simulink model "PosControl_Sim"  (R2016b)
settings: Solver=ode4  StartTime=0.0  StopTime=20  FixedStep=0.001  RelTol=1e-3
InitFcn:
  | Init_control;
values from neighbouring files (symbols this model uses):
  DEG2RAD = 0.0174533    [Init_control.m]
  Kd_PITCH_AgngleRate = 0.001    [Init_control.m]
  Kd_ROLL_AgngleRate = 0.001    [Init_control.m]
  Kd_YAW_AngleRate = 0.00    (= 0)    [Init_control.m]
  Ki_PITCH_AgngleRate = 0.02    [Init_control.m]
  Ki_ROLL_AgngleRate = 0.02    [Init_control.m]
  Ki_YAW_AngleRate = 0.01    [Init_control.m]
  Kp_PITCH_AgngleRate = 0.1    [Init_control.m]
  Kp_PITCH_ANGLE = 6.5    [Init_control.m]
  Kp_ROLL_AgngleRate = 0.1    [Init_control.m]
  Kp_ROLL_ANGLE = 6.5    [Init_control.m]
  Kp_YAW_AngleRate = 0.3    [Init_control.m]
  Kpxp = 1.2    [Init_control.m]
  Kpyp = 1.2    [Init_control.m]
  Kpzp = 4.0    (= 4)    [Init_control.m]
  Kvxd = 0.01    [Init_control.m]
  Kvxi = 0.4    [Init_control.m]
  Kvxp = 1.5    [Init_control.m]
  Kvyd = 0.01    [Init_control.m]
  Kvyi = 0.4    [Init_control.m]
  Kvyp = 1.5    [Init_control.m]
  Kvzd = 0.005    [Init_control.m]
  Kvzi = 0.01    [Init_control.m]
  Kvzp = 0.45    [Init_control.m]
  MAX_CONTROL_ANGLE_PITCH = 35    [Init_control.m]
  MAX_CONTROL_ANGLE_RATE_PITCH = 220    [Init_control.m]
  MAX_CONTROL_ANGLE_RATE_ROLL = 220    [Init_control.m]
  MAX_CONTROL_ANGLE_RATE_Y = 200    [Init_control.m]
  MAX_CONTROL_ANGLE_ROLL = 35    [Init_control.m]
  MAX_CONTROL_VELOCITY_XY = 5    [Init_control.m]
  MAX_CONTROL_VELOCITY_Z = 3    [Init_control.m]
  MAX_MAN_THR = 0.9    [Init_control.m]
  Saturation_I_ah = 3.43    [Init_control.m]
  Saturation_I_az = 5    [Init_control.m]
  Saturation_I_RP_Max = 0.3    [Init_control.m]
  Saturation_I_RP_Min = -0.3    [Init_control.m]
  Saturation_I_Y_Max = 0.2    [Init_control.m]
  Saturation_I_Y_Min = -0.2    [Init_control.m]
  THR_HOVER = 0.6085    [Init_control.m]
undefined symbols (not defined in the file or in its folder): DiscIntNeverNeededParam, earthRadius, ModelInit_RPM, ModelParam_envGravityAcc, ModelParam_motorCr, ModelParam_motorJm, ModelParam_motorT, ModelParam_motorWb, ModelParam_rotorCm, ModelParam_rotorCt, ModelParam_uavCd, ModelParam_uavJ, ModelParam_uavMass, ModelParam_uavR
libraries: simulink x7, aerolibutil x2, aerolibfltsims x2, aerolibtransform2 x1, aerolibanimutils x1
settings Model: Creator=dream  LastModifiedBy=Mr Wang
settings DebuggingCC: BusObjectLabelMismatch=error

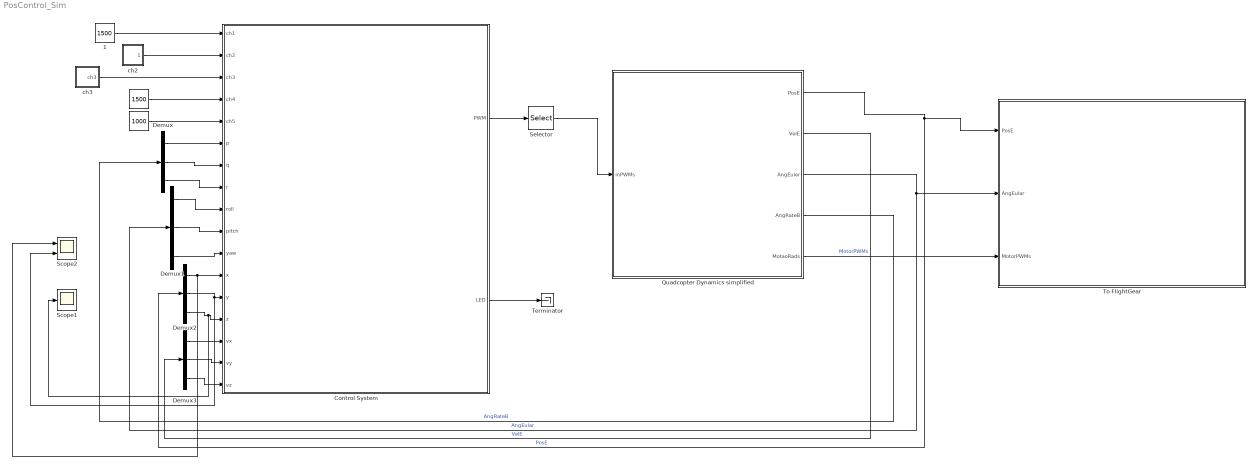
== system PosControl_Sim ==
  " " : Constant  Value=1000  OutDataTypeStr=uint16
  "          " : Constant  Value=1500  OutDataTypeStr=uint16
  "   1" : Constant  Value=1500  OutDataTypeStr=uint16
  Control System : Subsystem
      mask Display: image('icon\pixhawk.png');
  Demux{,1..3} (4 alike) : Demux  Outputs=3
  "Quadcopter Dynamics simplified " : Subsystem
      mask Display: image('./icon/F450.png');
  Scope1 : Scope
  Scope2 : Scope  NumInputPorts=2
  Selector : Selector  InputPortWidth=8  IndexOptions=Index vector (dialog)  Indices=[1:4]  OutputSizes=1
  Terminator : Terminator
  To FlightGear : Subsystem
      mask Display: image('./icon/FlightGear.png');
  ch2 : Subsystem
  ch3 : Subsystem
  wires:
  "Quadcopter Dynamics simplified "/1(PosE) -> To FlightGear/1(PosE), Demux2/1  "PosE"
  "Quadcopter Dynamics simplified "/5(MotaoRads) -> To FlightGear/3(MotorPWMs)  "MotorPWMs"
  Control System/2(LED) -> Terminator/1
  "Quadcopter Dynamics simplified "/3(AngEuler) -> To FlightGear/2(AngEular), Demux1/1  "AngEular"
  "          "/1 -> Control System/4(ch4)
  "Quadcopter Dynamics simplified "/4(AngRateB) -> Demux/1  "AngRateB"
  " "/1 -> Control System/5(ch5)
  Demux/1 -> Control System/6(p)
  Demux/2 -> Control System/7(q)
  Demux/3 -> Control System/8(r)
  Demux1/1 -> Control System/9(roll)
  Demux1/2 -> Control System/10(pitch)
  Demux1/3 -> Control System/11(yaw)
  Control System/1(PWM) -> Selector/1
  Demux2/1 -> Control System/12(x), Scope2/1
  Demux2/2 -> Scope2/2, Control System/13(y)
  Demux2/3 -> Scope1/1, Control System/14(z)
  Demux3/1 -> Control System/15(vx)
  Demux3/2 -> Control System/16(vy)
  Demux3/3 -> Control System/17(vz)
  "Quadcopter Dynamics simplified "/2(VelE) -> Demux3/1  "VelE"
  "   1"/1 -> Control System/1(ch1)
  ch2/1(ch2) -> Control System/2(ch2)
  ch3/1(ch3) -> Control System/3(ch3)
  Selector/1 -> "Quadcopter Dynamics simplified "/1(inPWMs)

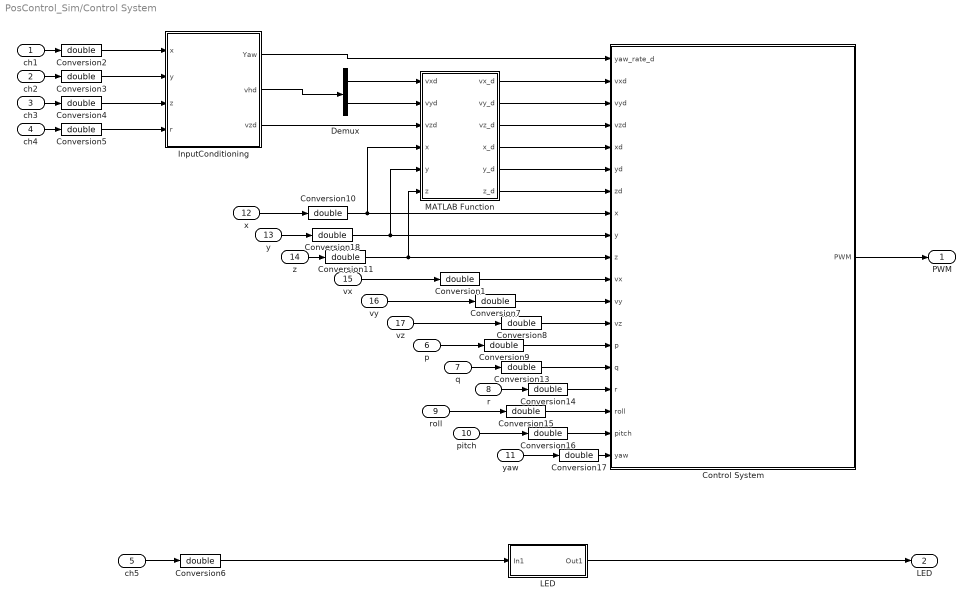
== system PosControl_Sim/Control System ==
  ch1 : Inport  OutDataTypeStr=uint16  PortDimensions=1
  ch2 : Inport  Port=2  OutDataTypeStr=uint16  PortDimensions=1
  ch3 : Inport  Port=3  OutDataTypeStr=uint16  PortDimensions=1
  ch4 : Inport  Port=4  OutDataTypeStr=uint16  PortDimensions=1
  ch5 : Inport  Port=5  OutDataTypeStr=uint16  PortDimensions=1  Interpolate=off
  p : Inport  Port=6  PortDimensions=1
  q : Inport  Port=7  PortDimensions=1
  r : Inport  Port=8  PortDimensions=1
  roll : Inport  Port=9  PortDimensions=1
  pitch : Inport  Port=10  PortDimensions=1
  yaw : Inport  Port=11  PortDimensions=1
  x : Inport  Port=12
  y : Inport  Port=13
  z : Inport  Port=14
  vx : Inport  Port=15
  vy : Inport  Port=16
  vz : Inport  Port=17
  Control System : Subsystem
  Conversion{1..11,13..18} (17 alike) : DataTypeConversion  OutDataTypeStr=double
  Demux : Demux  Outputs=2
  InputConditioning : Subsystem
  "LED " : Subsystem
  MATLAB Function : MATLAB Function  TreatAsAtomicUnit=on
  PWM : Outport  PortDimensions=8
  LED : Outport  Port=2  PortDimensions=1
  wires:
  ch3/1 -> Conversion4/1
  ch5/1 -> Conversion6/1
  InputConditioning/1(Yaw) -> Control System/1(yaw_rate_d)
  ch4/1 -> Conversion5/1
  "LED "/1(Out1) -> LED/1
  Conversion6/1 -> "LED "/1(In1)
  Conversion5/1 -> InputConditioning/4(r)
  Control System/1(PWM) -> PWM/1
  ch1/1 -> Conversion2/1
  ch2/1 -> Conversion3/1
  InputConditioning/2(vhd) -> Demux/1
  Demux/1 -> MATLAB Function/1(vxd)
  Demux/2 -> MATLAB Function/2(vyd)
  InputConditioning/3(vzd) -> MATLAB Function/3(vzd)
  y/1 -> Conversion18/1
  z/1 -> Conversion11/1
  vy/1 -> Conversion7/1
  MATLAB Function/4(x_d) -> Control System/5(xd)
  MATLAB Function/5(y_d) -> Control System/6(yd)
  MATLAB Function/6(z_d) -> Control System/7(zd)
  Conversion2/1 -> InputConditioning/1(x)
  Conversion3/1 -> InputConditioning/2(y)
  vx/1 -> Conversion1/1
  Conversion1/1 -> Control System/11(vx)
  Conversion7/1 -> Control System/12(vy)
  vz/1 -> Conversion8/1
  Conversion8/1 -> Control System/13(vz)
  Conversion18/1 -> MATLAB Function/5(y), Control System/9(y)
  Conversion11/1 -> MATLAB Function/6(z), Control System/10(z)
  MATLAB Function/1(vx_d) -> Control System/2(vxd)
  MATLAB Function/2(vy_d) -> Control System/3(vyd)
  MATLAB Function/3(vz_d) -> Control System/4(vzd)
  roll/1 -> Conversion15/1
  pitch/1 -> Conversion16/1
  p/1 -> Conversion9/1
  q/1 -> Conversion13/1
  r/1 -> Conversion14/1
  Conversion9/1 -> Control System/14(p)
  Conversion13/1 -> Control System/15(q)
  Conversion14/1 -> Control System/16(r)
  Conversion15/1 -> Control System/17(roll)
  Conversion16/1 -> Control System/18(pitch)
  yaw/1 -> Conversion17/1
  Conversion17/1 -> Control System/19(yaw)
  Conversion4/1 -> InputConditioning/3(z)
  x/1 -> Conversion10/1
  Conversion10/1 -> MATLAB Function/4(x), Control System/8(x)

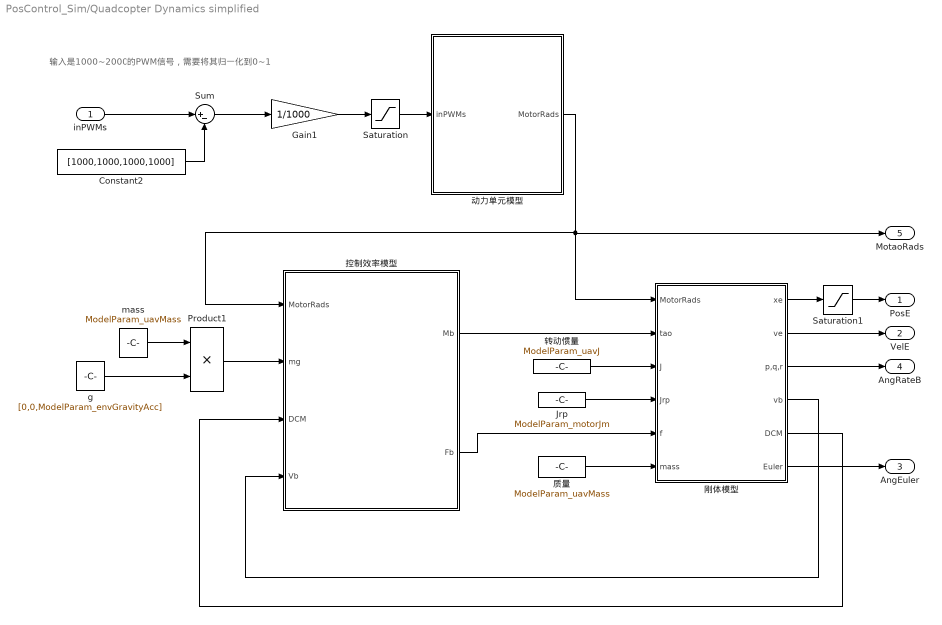
== system PosControl_Sim/Quadcopter Dynamics simplified  ==
  note: 输入是1000~2000的PWM信号，需要将其归一化到0~1
  inPWMs : Inport
  Constant2 : Constant  Value=[1000,1000,1000,1000]
  Gain1 : Gain  Gain=1/1000
  Jrp : Constant  Value=ModelParam_motorJm
  Product1 : Product
  Saturation : Saturate  UpperLimit=1  LowerLimit=0
  Saturation1 : Saturate  UpperLimit=[inf,inf,0]  LowerLimit=[-inf,-inf,-inf]
  Sum : Sum  Inputs=|+-
  g : Constant  Value=[0,0,ModelParam_envGravityAcc]
  mass : Constant  Value=ModelParam_uavMass
  刚体模型 : Subsystem
  动力单元模型 : Subsystem
  控制效率模型 : Subsystem
  质量 : Constant  Value=ModelParam_uavMass
  转动惯量 : Constant  Value=ModelParam_uavJ
  PosE : Outport
  VelE : Outport  Port=2
  AngEuler : Outport  Port=3
  AngRateB : Outport  Port=4
  MotaoRads : Outport  Port=5
  wires:
  g/1 -> Product1/2
  Constant2/1 -> Sum/2
  控制效率模型/2(Fb) -> 刚体模型/5(f)
  inPWMs/1 -> Sum/1
  控制效率模型/1(Mb) -> 刚体模型/2(tao)
  刚体模型/6(Euler) -> AngEuler/1
  Saturation1/1 -> PosE/1
  刚体模型/4("vb ") -> 控制效率模型/4(Vb)
  Product1/1 -> 控制效率模型/2(mg)
  Sum/1 -> Gain1/1
  刚体模型/2(ve) -> VelE/1
  Gain1/1 -> Saturation/1
  转动惯量/1 -> 刚体模型/3(J)
  动力单元模型/1(MotorRads) -> MotaoRads/1, 刚体模型/1(MotorRads), 控制效率模型/1(MotorRads)
  刚体模型/1("xe ") -> Saturation1/1
  刚体模型/5(DCM) -> 控制效率模型/3(DCM)
  mass/1 -> Product1/1
  质量/1 -> 刚体模型/6(mass)
  Jrp/1 -> 刚体模型/4(Jrp)
  刚体模型/3("p,q,r ") -> AngRateB/1
  Saturation/1 -> 动力单元模型/1(inPWMs)

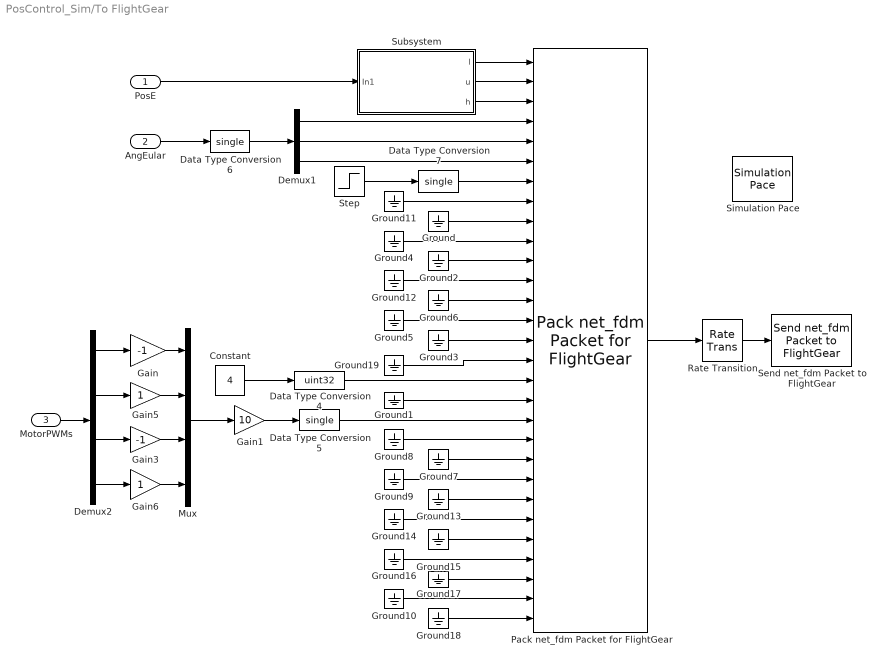
== system PosControl_Sim/To FlightGear ==
  PosE : Inport
  AngEular : Inport  Port=2
  MotorPWMs : Inport  Port=3
  Constant : Constant  Value=4
  Data Type Conversion4 : DataTypeConversion  OutDataTypeStr=uint32
  Data Type Conversion5 : DataTypeConversion  OutDataTypeStr=single
  Data Type Conversion6 : DataTypeConversion  OutDataTypeStr=single
  Data Type Conversion7 : DataTypeConversion  OutDataTypeStr=single
  Demux1 : Demux  Outputs=3
  Demux2 : Demux
  Gain : Gain  Gain=-1
  Gain1 : Gain  Gain=10
  Gain3 : Gain  Gain=-1
  Gain5 : Gain
  Gain6 : Gain
  Ground{,1..19} (20 alike) : Ground
  Mux : Mux
  Pack net_fdm Packet for FlightGear : aerolibfltsims/Pack net_fdm Packet for FlightGear  FlightGearVersion=v2016.1  ShowPositionAttitudeInputs=on  ShowVelocityAccelerationInputs=off  ShowControlSurfacePositionInputs=on  ShowEngineFuelInputs=on  ShowLandingGearInputs=off  ShowEnvironmentInputs=off  SampleTime=0.01
  Rate Transition : RateTransition
  Send net_fdm Packet to FlightGear : aerolibfltsims/Send net_fdm Packet to FlightGear  DestinationIpAddress=127.0.0.1  DestinationPort=5502  LocalIpPort=-1  varLen=off  SampleTime=0.005
  Simulation Pace : aerolibanimutils/Simulation Pace  SimulationPace=1  SleepMode=MATLAB Thread  OutputPaceError=off  SampleTime=-1
      settings: AttributesFormatString=%<SimulationPace> sec/sec
  Step : Step  Time=5  SampleTime=0
  Subsystem : Subsystem
  wires:
  Pack net_fdm Packet for FlightGear/1 -> Rate Transition/1
  Data Type Conversion7/1 -> Pack net_fdm Packet for FlightGear/7
  Ground8/1 -> Pack net_fdm Packet for FlightGear/20
  Ground/1 -> Pack net_fdm Packet for FlightGear/9
  Ground7/1 -> Pack net_fdm Packet for FlightGear/21
  Ground9/1 -> Pack net_fdm Packet for FlightGear/22
  Ground13/1 -> Pack net_fdm Packet for FlightGear/23
  Ground14/1 -> Pack net_fdm Packet for FlightGear/24
  Ground15/1 -> Pack net_fdm Packet for FlightGear/25
  Ground16/1 -> Pack net_fdm Packet for FlightGear/26
  Ground17/1 -> Pack net_fdm Packet for FlightGear/27
  Ground10/1 -> Pack net_fdm Packet for FlightGear/28
  Ground18/1 -> Pack net_fdm Packet for FlightGear/29
  Step/1 -> Data Type Conversion7/1
  Data Type Conversion4/1 -> Pack net_fdm Packet for FlightGear/17
  Ground1/1 -> Pack net_fdm Packet for FlightGear/18
  Ground3/1 -> Pack net_fdm Packet for FlightGear/15
  Ground5/1 -> Pack net_fdm Packet for FlightGear/14
  Ground6/1 -> Pack net_fdm Packet for FlightGear/13
  Ground4/1 -> Pack net_fdm Packet for FlightGear/10
  Ground11/1 -> Pack net_fdm Packet for FlightGear/8
  Constant/1 -> Data Type Conversion4/1
  Data Type Conversion5/1 -> Pack net_fdm Packet for FlightGear/19
  Ground2/1 -> Pack net_fdm Packet for FlightGear/11
  Ground12/1 -> Pack net_fdm Packet for FlightGear/12
  AngEular/1 -> Data Type Conversion6/1
  MotorPWMs/1 -> Demux2/1
  Mux/1 -> Gain1/1
  Demux2/1 -> Gain/1
  Demux2/3 -> Gain3/1
  Gain/1 -> Mux/1
  Gain3/1 -> Mux/3
  Demux2/2 -> Gain5/1
  Gain5/1 -> Mux/2
  Demux2/4 -> Gain6/1
  Gain6/1 -> Mux/4
  Rate Transition/1 -> Send net_fdm Packet to FlightGear/1
  PosE/1 -> Subsystem/1(In1)
  Subsystem/1("l ") -> Pack net_fdm Packet for FlightGear/1
  Subsystem/2(u) -> Pack net_fdm Packet for FlightGear/2
  Subsystem/3(h) -> Pack net_fdm Packet for FlightGear/3
  Ground19/1 -> Pack net_fdm Packet for FlightGear/16
  Demux1/1 -> Pack net_fdm Packet for FlightGear/4
  Demux1/2 -> Pack net_fdm Packet for FlightGear/5
  Demux1/3 -> Pack net_fdm Packet for FlightGear/6
  Data Type Conversion6/1 -> Demux1/1
  Gain1/1 -> Data Type Conversion5/1

== system PosControl_Sim/ch2 ==
  "   " : Constant  Value=1500  OutDataTypeStr=uint16
  Constant1 : Constant  Value=200
  Constant2 : Constant  Value=200
  Data Type Conversion1 : DataTypeConversion  OutDataTypeStr=uint16
  Data Type Conversion2 : DataTypeConversion  OutDataTypeStr=uint16
  Delay1 : Delay  DelayLength=5000
  Delay2 : Delay  DelayLength=15000
  Sum1 : Sum  Inputs=|++-
  ch2 : Outport
  wires:
  Sum1/1 -> ch2/1
  Data Type Conversion1/1 -> Delay1/1
  Delay2/1 -> Sum1/3
  Constant2/1 -> Data Type Conversion2/1
  Data Type Conversion2/1 -> Delay2/1
  "   "/1 -> Sum1/1
  Delay1/1 -> Sum1/2
  Constant1/1 -> Data Type Conversion1/1

== system PosControl_Sim/ch3 ==
  "  " : Constant  Value=1700  OutDataTypeStr=uint16
  Constant : Constant  Value=200
  Data Type Conversion : DataTypeConversion  OutDataTypeStr=uint16
  Delay : Delay  DelayLength=4500
  Sum : Sum  Inputs=|+-
  ch3 : Outport
  wires:
  Sum/1 -> ch3/1
  "  "/1 -> Sum/1
  Constant/1 -> Data Type Conversion/1
  Delay/1 -> Sum/2
  Data Type Conversion/1 -> Delay/1

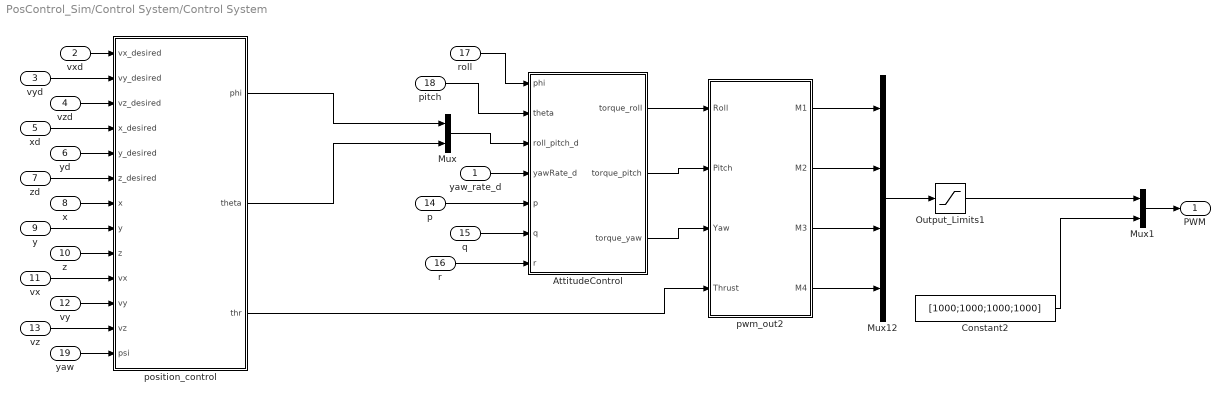
== system PosControl_Sim/Control System/Control System ==
  yaw_rate_d : Inport
  vxd : Inport  Port=2
  vyd : Inport  Port=3
  vzd : Inport  Port=4
  xd : Inport  Port=5
  yd : Inport  Port=6
  zd : Inport  Port=7
  x : Inport  Port=8
  y : Inport  Port=9
  z : Inport  Port=10
  vx : Inport  Port=11
  vy : Inport  Port=12
  vz : Inport  Port=13
  p : Inport  Port=14  PortDimensions=1
  q : Inport  Port=15  PortDimensions=1
  r : Inport  Port=16  PortDimensions=1
  roll : Inport  Port=17  PortDimensions=1
  pitch : Inport  Port=18  PortDimensions=1
  yaw : Inport  Port=19
  AttitudeControl : Subsystem
  Constant2 : Constant  Value=[1000;1000;1000;1000]
  Mux : Mux  Inputs=2
  Mux1 : Mux  Inputs=2
  Mux12 : Mux
  Output_Limits1 : Saturate  UpperLimit=2000  LowerLimit=1000
  position_control : Subsystem
  pwm_out2 : MATLAB Function  SystemSampleTime=0.004
  PWM : Outport  PortDimensions=8
  wires:
  pitch/1 -> AttitudeControl/2(theta)
  q/1 -> AttitudeControl/6(q)
  roll/1 -> AttitudeControl/1(phi)
  r/1 -> AttitudeControl/7(r)
  p/1 -> AttitudeControl/5(p)
  Mux/1 -> AttitudeControl/3(roll_pitch_d)
  position_control/1(phi) -> Mux/1
  vy/1 -> position_control/11(vy)
  vx/1 -> position_control/10(vx)
  vxd/1 -> position_control/1(vx_desired)
  y/1 -> position_control/8(y)
  vzd/1 -> position_control/3(vz_desired)
  x/1 -> position_control/7(x)
  z/1 -> position_control/9(z)
  vz/1 -> position_control/12(vz)
  yaw_rate_d/1 -> AttitudeControl/4(yawRate_d)
  xd/1 -> position_control/4(x_desired)
  yd/1 -> position_control/5(y_desired)
  vyd/1 -> position_control/2(vy_desired)
  zd/1 -> position_control/6(z_desired)
  yaw/1 -> position_control/13(psi)
  position_control/2(theta) -> Mux/2
  Mux12/1 -> Output_Limits1/1
  pwm_out2/1(M1) -> Mux12/1
  pwm_out2/3(M3) -> Mux12/3
  pwm_out2/2(M2) -> Mux12/2
  pwm_out2/4(M4) -> Mux12/4
  Constant2/1 -> Mux1/2
  Output_Limits1/1 -> Mux1/1
  Mux1/1 -> PWM/1
  AttitudeControl/1(torque_roll) -> pwm_out2/1(Roll)
  AttitudeControl/2(torque_pitch) -> pwm_out2/2(Pitch)
  AttitudeControl/3(torque_yaw) -> pwm_out2/3(Yaw)
  position_control/3(thr) -> pwm_out2/4(Thrust)

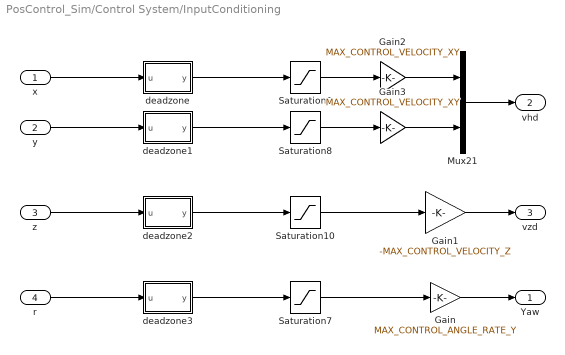
== system PosControl_Sim/Control System/InputConditioning ==
  x : Inport
  y : Inport  Port=2
  z : Inport  Port=3
  r : Inport  Port=4
  Gain : Gain  Gain=MAX_CONTROL_ANGLE_RATE_Y
  Gain1 : Gain  Gain=-MAX_CONTROL_VELOCITY_Z  OutDataTypeStr=Inherit: Inherit via back propagation
  Gain2 : Gain  Gain=MAX_CONTROL_VELOCITY_XY  OutDataTypeStr=Inherit: Inherit via back propagation
  Gain3 : Gain  Gain=MAX_CONTROL_VELOCITY_XY  OutDataTypeStr=Inherit: Inherit via back propagation
  Mux21 : Mux  Inputs=2
  Saturation{7..10} (4 alike) : Saturate  UpperLimit=1  LowerLimit=-1
  deadzone : MATLAB Function  TreatAsAtomicUnit=on
  deadzone1 : MATLAB Function  TreatAsAtomicUnit=on
  deadzone2 : MATLAB Function  TreatAsAtomicUnit=on
  deadzone3 : MATLAB Function  TreatAsAtomicUnit=on
  Yaw : Outport
  vhd : Outport  Port=2
  vzd : Outport  Port=3
  wires:
  Saturation10/1 -> Gain1/1
  Saturation7/1 -> Gain/1
  Saturation8/1 -> Gain3/1
  deadzone2/1(y) -> Saturation10/1
  deadzone/1(y) -> Saturation9/1
  deadzone1/1(y) -> Saturation8/1
  Saturation9/1 -> Gain2/1
  deadzone3/1(y) -> Saturation7/1
  y/1 -> deadzone1/1(u)
  z/1 -> deadzone2/1(u)
  x/1 -> deadzone/1(u)
  r/1 -> deadzone3/1(u)
  Gain/1 -> Yaw/1
  Gain1/1 -> vzd/1
  Mux21/1 -> vhd/1
  Gain2/1 -> Mux21/1
  Gain3/1 -> Mux21/2

== system PosControl_Sim/Control System/LED  ==
  In1 : Inport
  Compare To Constant3 : simulink/Logic and Bit Operations/Compare To Constant  relop=>=  const=uint16(1500)  OutDataTypeStr=boolean
  Out1 : Outport
  wires:
  Compare To Constant3/1 -> Out1/1
  In1/1 -> Compare To Constant3/1

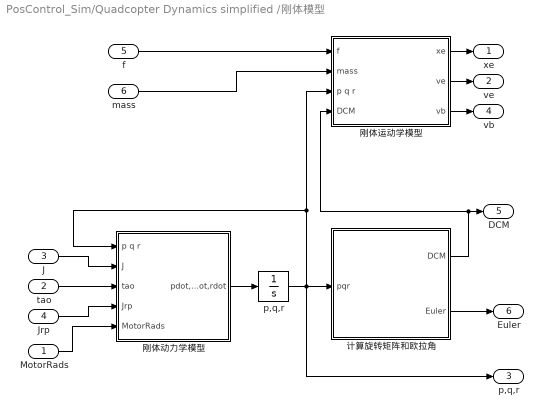
== system PosControl_Sim/Quadcopter Dynamics simplified /刚体模型 ==
  MotorRads : Inport
  tao : Inport  Port=2
  J : Inport  Port=3
  Jrp : Inport  Port=4
  f : Inport  Port=5
  mass : Inport  Port=6
  p,q,r : Integrator
  刚体动力学模型 : Subsystem
  刚体运动学模型 : Subsystem
  计算旋转矩阵和欧拉角 : Subsystem
  "xe " : Outport
  ve : Outport  Port=2
  "p,q,r " : Outport  Port=3
  "vb " : Outport  Port=4
  DCM : Outport  Port=5
  Euler : Outport  Port=6
  wires:
  J/1 -> 刚体动力学模型/2(J)
  tao/1 -> 刚体动力学模型/3(tao)
  Jrp/1 -> 刚体动力学模型/4(Jrp)
  MotorRads/1 -> 刚体动力学模型/5(MotorRads)
  刚体动力学模型/1(pdot,qdot,rdot) -> p,q,r/1
  计算旋转矩阵和欧拉角/1(DCM) -> DCM/1, 刚体运动学模型/4(DCM)
  计算旋转矩阵和欧拉角/2(Euler) -> Euler/1
  f/1 -> 刚体运动学模型/1(f)
  mass/1 -> 刚体运动学模型/2(mass)
  刚体运动学模型/1("xe ") -> "xe "/1
  刚体运动学模型/2(ve) -> ve/1
  p,q,r/1 -> 刚体运动学模型/3(p q r), 刚体动力学模型/1(p q r), "p,q,r "/1, 计算旋转矩阵和欧拉角/1(pqr)
  刚体运动学模型/3("vb ") -> "vb "/1

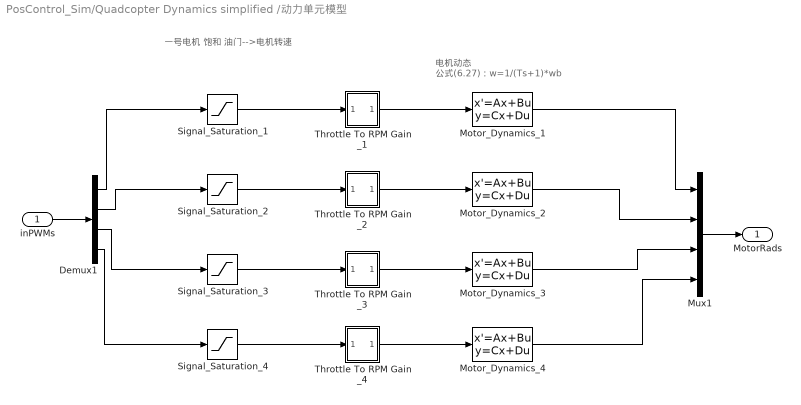
== system PosControl_Sim/Quadcopter Dynamics simplified /动力单元模型 ==
  note: 一号电机
      |
      |              饱和                             油门-->电机转速
  note: 电机动态
      | 公式(6.27)：w=1/(Ts+1)*wb
  inPWMs : Inport
  Demux1 : Demux
  Motor_Dynamics_{1..4} (4 alike) : StateSpace  A=-1/ModelParam_motorT  C=1/ModelParam_motorT  D=0  X0=ModelInit_RPM*ModelParam_motorT
  Mux1 : Mux
  Signal_Saturation_{1..4} (4 alike) : Saturate  UpperLimit=1  LowerLimit=0
  Throttle To RPM Gain _1 : Subsystem
  Throttle To RPM Gain _2 : Subsystem
  Throttle To RPM Gain _3 : Subsystem
  Throttle To RPM Gain _4 : Subsystem
  MotorRads : Outport
  wires:
  Demux1/1 -> Signal_Saturation_1/1
  Demux1/2 -> Signal_Saturation_2/1
  Demux1/3 -> Signal_Saturation_3/1
  Demux1/4 -> Signal_Saturation_4/1
  inPWMs/1 -> Demux1/1
  Throttle To RPM Gain _1/1(Out5) -> Motor_Dynamics_1/1
  Throttle To RPM Gain _2/1(Out5) -> Motor_Dynamics_2/1
  Throttle To RPM Gain _3/1(Out5) -> Motor_Dynamics_3/1
  Mux1/1 -> MotorRads/1
  Signal_Saturation_1/1 -> Throttle To RPM Gain _1/1(In5)
  Motor_Dynamics_1/1 -> Mux1/1
  Motor_Dynamics_2/1 -> Mux1/2
  Motor_Dynamics_3/1 -> Mux1/3
  Motor_Dynamics_4/1 -> Mux1/4
  Signal_Saturation_2/1 -> Throttle To RPM Gain _2/1(In5)
  Signal_Saturation_3/1 -> Throttle To RPM Gain _3/1(In5)
  Signal_Saturation_4/1 -> Throttle To RPM Gain _4/1(In5)
  Throttle To RPM Gain _4/1(Out5) -> Motor_Dynamics_4/1

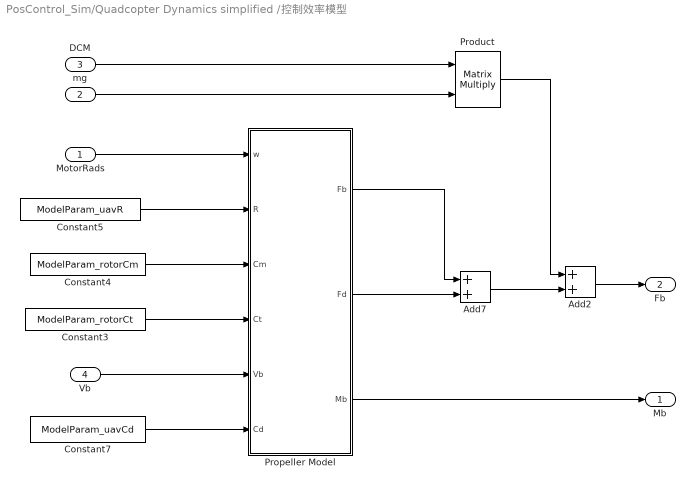
== system PosControl_Sim/Quadcopter Dynamics simplified /控制效率模型 ==
  MotorRads : Inport
  mg : Inport  Port=2
  DCM : Inport  Port=3
  Vb : Inport  Port=4
  Add2 : Sum
  Add7 : Sum
  Constant3 : Constant  Value=ModelParam_rotorCt
  Constant4 : Constant  Value=ModelParam_rotorCm
  Constant5 : Constant  Value=ModelParam_uavR
  Constant7 : Constant  Value=ModelParam_uavCd
  Product : Product  Multiplication=Matrix(*)
  Propeller Model : MATLAB Function  TreatAsAtomicUnit=on
  Mb : Outport
  Fb : Outport  Port=2
  wires:
  MotorRads/1 -> Propeller Model/1(w)
  Constant4/1 -> Propeller Model/3(Cm)
  Constant5/1 -> Propeller Model/2(R)
  Vb/1 -> Propeller Model/5(Vb)
  Constant7/1 -> Propeller Model/6(Cd)
  DCM/1 -> Product/1
  mg/1 -> Product/2
  Product/1 -> Add2/1
  Propeller Model/1(Fb) -> Add7/1
  Add7/1 -> Add2/2
  Propeller Model/2(Fd) -> Add7/2
  Constant3/1 -> Propeller Model/4(Ct)
  Add2/1 -> Fb/1
  Propeller Model/3(Mb) -> Mb/1

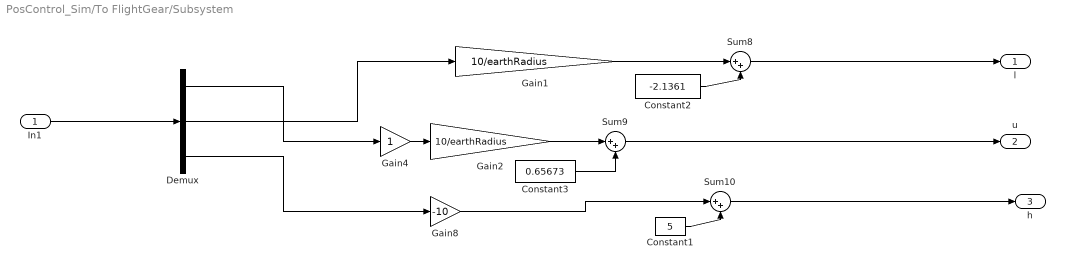
== system PosControl_Sim/To FlightGear/Subsystem ==
  In1 : Inport
  Constant1 : Constant  Value=5  VectorParams1D=off
  Constant2 : Constant  Value=-2.1361  VectorParams1D=off
  Constant3 : Constant  Value=0.65673  VectorParams1D=off
  Demux : Demux  Outputs=3
  Gain1 : Gain  Gain=10/earthRadius
  Gain2 : Gain  Gain=10/earthRadius
  Gain4 : Gain
  Gain8 : Gain  Gain=-10
  Sum10 : Sum  Inputs=|++
  Sum8 : Sum  Inputs=|++
  Sum9 : Sum  Inputs=|++
  "l " : Outport
  u : Outport  Port=2
  h : Outport  Port=3
  wires:
  Constant3/1 -> Sum9/2
  Constant1/1 -> Sum10/2
  Demux/1 -> Gain4/1
  Demux/3 -> Gain8/1
  Constant2/1 -> Sum8/2
  Gain2/1 -> Sum9/1
  Gain1/1 -> Sum8/1
  Gain8/1 -> Sum10/1
  Demux/2 -> Gain1/1
  Gain4/1 -> Gain2/1
  Sum10/1 -> h/1
  Sum9/1 -> u/1
  In1/1 -> Demux/1
  Sum8/1 -> "l "/1

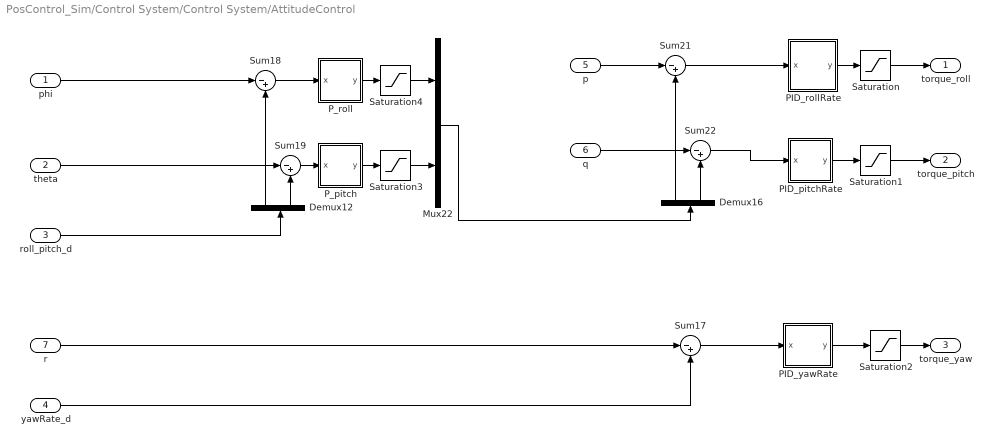
== system PosControl_Sim/Control System/Control System/AttitudeControl ==
  phi : Inport
  theta : Inport  Port=2
  roll_pitch_d : Inport  Port=3
  yawRate_d : Inport  Port=4
  p : Inport  Port=5
  q : Inport  Port=6
  r : Inport  Port=7
  Demux12 : Demux  Outputs=2
  Demux16 : Demux  Outputs=2
  Mux22 : Mux  Inputs=2
  PID_pitchRate : Subsystem
  PID_rollRate : Subsystem
  PID_yawRate : Subsystem
  "P_pitch " : Subsystem
  "P_roll " : Subsystem
  Saturation : Saturate  UpperLimit=1  LowerLimit=-1
  Saturation1 : Saturate  UpperLimit=1  LowerLimit=-1
  Saturation2 : Saturate
  Saturation3 : Saturate  UpperLimit=MAX_CONTROL_ANGLE_RATE_PITCH  LowerLimit=-MAX_CONTROL_ANGLE_RATE_PITCH
  Saturation4 : Saturate  UpperLimit=MAX_CONTROL_ANGLE_RATE_ROLL  LowerLimit=-MAX_CONTROL_ANGLE_RATE_ROLL
  Sum{17..19,21..22} (5 alike) : Sum  Inputs=|-+
  torque_roll : Outport
  torque_pitch : Outport  Port=2
  torque_yaw : Outport  Port=3
  wires:
  r/1 -> Sum17/1
  Sum19/1 -> "P_pitch "/1(x)
  "P_pitch "/1(y) -> Saturation3/1
  "P_roll "/1(y) -> Saturation4/1
  roll_pitch_d/1 -> Demux12/1
  Demux12/1 -> Sum18/2
  Demux12/2 -> Sum19/2
  phi/1 -> Sum18/1
  theta/1 -> Sum19/1
  Sum18/1 -> "P_roll "/1(x)
  Sum22/1 -> PID_pitchRate/1(x)
  Sum17/1 -> PID_yawRate/1(x)
  p/1 -> Sum21/1
  q/1 -> Sum22/1
  Sum21/1 -> PID_rollRate/1(x)
  Demux16/1 -> Sum21/2
  PID_pitchRate/1(y) -> Saturation1/1
  PID_rollRate/1(y) -> Saturation/1
  PID_yawRate/1(y) -> Saturation2/1
  yawRate_d/1 -> Sum17/2
  Saturation/1 -> torque_roll/1
  Saturation1/1 -> torque_pitch/1
  Saturation2/1 -> torque_yaw/1
  Mux22/1 -> Demux16/1
  Saturation4/1 -> Mux22/1
  Saturation3/1 -> Mux22/2
  Demux16/2 -> Sum22/2

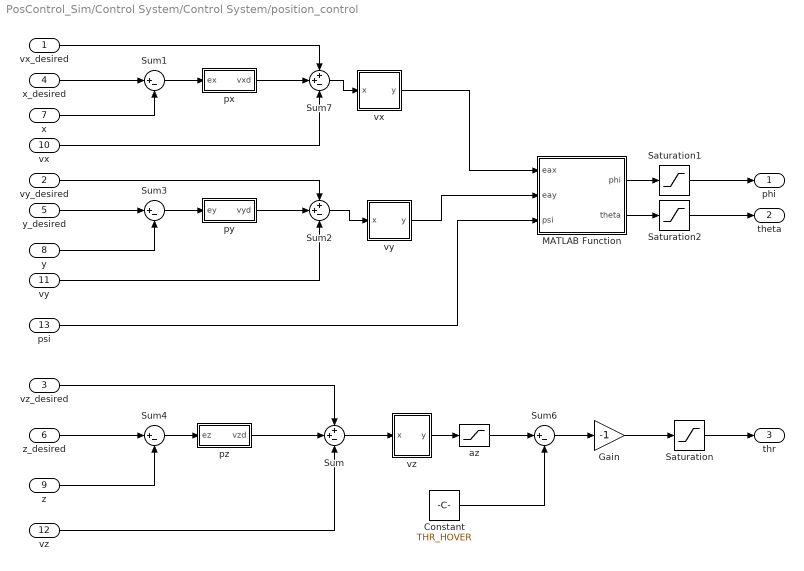
== system PosControl_Sim/Control System/Control System/position_control ==
  vx_desired : Inport
  vy_desired : Inport  Port=2
  vz_desired : Inport  Port=3
  x_desired : Inport  Port=4
  y_desired : Inport  Port=5
  z_desired : Inport  Port=6
  x : Inport  Port=7
  y : Inport  Port=8
  z : Inport  Port=9
  vx : Inport  Port=10
  vy : Inport  Port=11
  vz : Inport  Port=12
  psi : Inport  Port=13
  Constant : Constant  Value=THR_HOVER
  Gain : Gain  Gain=-1
  MATLAB Function : MATLAB Function  TreatAsAtomicUnit=on
  Saturation : Saturate  UpperLimit=MAX_MAN_THR  LowerLimit=0
  Saturation1 : Saturate  UpperLimit=MAX_CONTROL_ANGLE_ROLL*DEG2RAD  LowerLimit=-MAX_CONTROL_ANGLE_ROLL*DEG2RAD
  Saturation2 : Saturate  UpperLimit=MAX_CONTROL_ANGLE_PITCH*DEG2RAD  LowerLimit=-MAX_CONTROL_ANGLE_PITCH*DEG2RAD
  Sum : Sum  Inputs=++-
  Sum{1,3..4,6} (4 alike) : Sum  Inputs=|+-
  Sum2 : Sum  Inputs=++-
  Sum7 : Sum  Inputs=++-
  az : Saturate  UpperLimit=0.4  LowerLimit=-0.4
  px : Subsystem
  py : Subsystem
  pz : Subsystem
  "vx " : Subsystem
  "vy " : Subsystem
  "vz " : Subsystem
  phi : Outport
  theta : Outport  Port=2
  thr : Outport  Port=3
  wires:
  Saturation/1 -> thr/1
  Gain/1 -> Saturation/1
  Sum6/1 -> Gain/1
  "vz "/1(y) -> az/1
  Sum4/1 -> pz/1(ez)
  z/1 -> Sum4/2
  Constant/1 -> Sum6/2
  Sum/1 -> "vz "/1(x)
  vz/1 -> Sum/3
  x/1 -> Sum1/2
  y/1 -> Sum3/2
  Sum3/1 -> py/1(ey)
  y_desired/1 -> Sum3/1
  vy/1 -> Sum2/3
  Sum2/1 -> "vy "/1(x)
  Sum7/1 -> "vx "/1(x)
  Sum1/1 -> px/1(ex)
  vy_desired/1 -> Sum2/1
  pz/1(vzd) -> Sum/2
  z_desired/1 -> Sum4/1
  vz_desired/1 -> Sum/1
  Saturation1/1 -> phi/1
  Saturation2/1 -> theta/1
  psi/1 -> MATLAB Function/3(psi)
  py/1(vyd) -> Sum2/2
  MATLAB Function/1(phi) -> Saturation1/1
  MATLAB Function/2(theta) -> Saturation2/1
  "vx "/1(y) -> MATLAB Function/1(eax)
  "vy "/1(y) -> MATLAB Function/2(eay)
  az/1 -> Sum6/1
  vx_desired/1 -> Sum7/1
  x_desired/1 -> Sum1/1
  vx/1 -> Sum7/3
  px/1(vxd) -> Sum7/2

== system PosControl_Sim/Quadcopter Dynamics simplified /刚体模型/刚体动力学模型 ==
  p q r : Inport
  J : Inport  Port=2
  tao : Inport  Port=3
  Jrp : Inport  Port=4
  MotorRads : Inport  Port=5
  Constant : Constant  Value=eye(3)
  Divide : Product  Inputs=*/  Multiplication=Matrix(*)
  J*w : Subsystem
  Product : Product  Multiplication=Matrix(*)
  Reshape1 : Reshape  OutputDimensionality=Column vector (2-D)
  Sum : Sum  Inputs=3
  wx(Jw) : aerolibutil/3x3 Cross Product
  陀螺力矩 : MATLAB Function  TreatAsAtomicUnit=on
  pdot,qdot,rdot : Outport
  wires:
  wx(Jw)/1 -> Sum/3
  MotorRads/1 -> 陀螺力矩/2(MotorRads)
  Jrp/1 -> 陀螺力矩/1(Jrp)
  tao/1 -> Sum/1
  J*w/1("J*w ") -> wx(Jw)/2
  p q r/1 -> wx(Jw)/1, 陀螺力矩/3(pqr), J*w/1(p q r)
  J/1 -> J*w/2(J), Divide/2
  Sum/1 -> Reshape1/1
  Divide/1 -> Product/1
  陀螺力矩/1(Ga) -> Sum/2
  Constant/1 -> Divide/1
  Reshape1/1 -> Product/2
  Product/1 -> pdot,qdot,rdot/1

== system PosControl_Sim/Quadcopter Dynamics simplified /刚体模型/刚体运动学模型 ==
  f : Inport
  mass : Inport  Port=2
  p q r : Inport  Port=3
  DCM : Inport  Port=4
  Product1 : Product  Multiplication=Matrix(*)
  Sum : Sum  Inputs=|+-
  Transpose : Math  Operator=transpose  SaturateOnIntegerOverflow=on
  Vbxw : aerolibutil/3x3 Cross Product
  a=f/m : Product  Inputs=*/
  vb : Integrator
  xe : Integrator
  "xe " : Outport
  ve : Outport  Port=2
  "vb " : Outport  Port=3
  wires:
  DCM/1 -> Transpose/1
  p q r/1 -> Vbxw/1
  f/1 -> a=f/m/1
  Vbxw/1 -> Sum/2
  mass/1 -> a=f/m/2
  Transpose/1 -> Product1/1
  Product1/1 -> ve/1, xe/1
  xe/1 -> "xe "/1
  Sum/1 -> vb/1
  a=f/m/1 -> Sum/1
  vb/1 -> Vbxw/2, "vb "/1, Product1/2

== system PosControl_Sim/Quadcopter Dynamics simplified /刚体模型/计算旋转矩阵和欧拉角 ==
  note: 四元数归一化
  note: 式（5.52）
  pqr : Inport
  Constant : Constant  Value=[1,0,0,0]
  Divide : Product  Inputs=*/
  Dot Product : DotProduct  InputSameDT=on  OutDataTypeStr=Inherit: Inherit via internal rule
  q : Integrator  InitialConditionSource=external
  四元数转DCM : aerolibtransform2/Quaternions to  Direction Cosine Matrix
  四元数转欧拉角 : MATLAB Function
  基于四元数模型 : MATLAB Function  TreatAsAtomicUnit=on
  DCM : Outport
  Euler : Outport  Port=2
  wires:
  Constant/1 -> q/2
  基于四元数模型/1(qdot) -> q/1
  q/1 -> Divide/1, Dot Product/2, Dot Product/1
  pqr/1 -> 基于四元数模型/1(pqr)
  四元数转DCM/1 -> DCM/1
  Dot Product/1 -> Divide/2
  Divide/1 -> 四元数转欧拉角/1(q), 基于四元数模型/2(q), 四元数转DCM/1
  四元数转欧拉角/1(y) -> Euler/1

== system PosControl_Sim/Quadcopter Dynamics simplified /动力单元模型/Throttle To RPM Gain _1 ==
  In5 : Inport
  Constant : Constant  Value=ModelParam_motorWb
  Gain : Gain  Gain=ModelParam_motorCr
  Sum1 : Sum  Inputs=++|
  Out5 : Outport
  wires:
  Sum1/1 -> Out5/1
  In5/1 -> Gain/1
  Gain/1 -> Sum1/2
  Constant/1 -> Sum1/1

== system PosControl_Sim/Quadcopter Dynamics simplified /动力单元模型/Throttle To RPM Gain _2 ==
  In5 : Inport
  Constant : Constant  Value=ModelParam_motorWb
  Gain : Gain  Gain=ModelParam_motorCr
  Sum1 : Sum  Inputs=++|
  Out5 : Outport
  wires:
  Constant/1 -> Sum1/1
  Gain/1 -> Sum1/2
  In5/1 -> Gain/1
  Sum1/1 -> Out5/1

== system PosControl_Sim/Quadcopter Dynamics simplified /动力单元模型/Throttle To RPM Gain _3 ==
  In5 : Inport
  Constant : Constant  Value=ModelParam_motorWb
  Gain : Gain  Gain=ModelParam_motorCr
  Sum1 : Sum  Inputs=++|
  Out5 : Outport
  wires:
  Sum1/1 -> Out5/1
  In5/1 -> Gain/1
  Gain/1 -> Sum1/2
  Constant/1 -> Sum1/1

== system PosControl_Sim/Quadcopter Dynamics simplified /动力单元模型/Throttle To RPM Gain _4 ==
  In5 : Inport
  Constant : Constant  Value=ModelParam_motorWb
  Gain : Gain  Gain=ModelParam_motorCr
  Sum1 : Sum  Inputs=++|
  Out5 : Outport
  wires:
  Constant/1 -> Sum1/1
  Gain/1 -> Sum1/2
  In5/1 -> Gain/1
  Sum1/1 -> Out5/1

== system PosControl_Sim/Control System/Control System/AttitudeControl/PID_pitchRate ==
  x : Inport
  Derivative Gain : Gain  DisableCoverage=on  Gain=Kd_PITCH_AgngleRate  ParamMin=-100  ParamMax=100  OutMin=-100  OutMax=100
  Discrete Derivative : simulink/Discrete/Discrete Derivative  gainval=1.0  ICPrevScaledInput=0.0  OutMin=[]  OutMax=[]  OutDataType=fixdt(1, 16)  OutScaling=2^-10  DoSatur=off
  Discrete-Time Integrator : DiscreteIntegrator  InitialConditionSetting=State (most efficient)  SampleTime=-1  LimitOutput=on  UpperSaturationLimit=Saturation_I_RP_Max  LowerSaturationLimit=Saturation_I_RP_Min  ICPrevOutput=DiscIntNeverNeededParam  ICPrevScaledInput=DiscIntNeverNeededParam
  Gain : Gain  Gain=Kp_PITCH_AgngleRate
  Integral Gain : Gain  DisableCoverage=on  Gain=Ki_PITCH_AgngleRate
  Sum : Sum  Inputs=+++
  y : Outport  InitialOutput=0
  wires:
  Discrete-Time Integrator/1 -> Sum/2
  Discrete Derivative/1 -> Sum/3
  Sum/1 -> y/1
  Gain/1 -> Sum/1
  Derivative Gain/1 -> Discrete Derivative/1
  Integral Gain/1 -> Discrete-Time Integrator/1
  x/1 -> Derivative Gain/1, Integral Gain/1, Gain/1

== system PosControl_Sim/Control System/Control System/AttitudeControl/PID_rollRate ==
  x : Inport
  Derivative Gain : Gain  DisableCoverage=on  Gain=Kd_ROLL_AgngleRate  ParamMin=-100  ParamMax=100  OutMin=-100  OutMax=100
  Discrete Derivative : simulink/Discrete/Discrete Derivative  gainval=1.0  ICPrevScaledInput=0.0  OutMin=[]  OutMax=[]  OutDataType=fixdt(1, 16)  OutScaling=2^-10  DoSatur=off
  Discrete-Time Integrator : DiscreteIntegrator  InitialConditionSetting=State (most efficient)  SampleTime=-1  LimitOutput=on  UpperSaturationLimit=Saturation_I_RP_Max  LowerSaturationLimit=Saturation_I_RP_Min  ICPrevOutput=DiscIntNeverNeededParam  ICPrevScaledInput=DiscIntNeverNeededParam
  Gain : Gain  Gain=Kp_ROLL_AgngleRate
  Integral Gain : Gain  DisableCoverage=on  Gain=Ki_ROLL_AgngleRate
  Sum : Sum  Inputs=+++
  y : Outport  InitialOutput=0
  wires:
  x/1 -> Gain/1, Integral Gain/1, Derivative Gain/1
  Integral Gain/1 -> Discrete-Time Integrator/1
  Derivative Gain/1 -> Discrete Derivative/1
  Gain/1 -> Sum/1
  Sum/1 -> y/1
  Discrete Derivative/1 -> Sum/3
  Discrete-Time Integrator/1 -> Sum/2

== system PosControl_Sim/Control System/Control System/AttitudeControl/PID_yawRate ==
  x : Inport
  Derivative Gain : Gain  DisableCoverage=on  Gain=Kd_YAW_AngleRate  ParamMin=-100  ParamMax=100  OutMin=-100  OutMax=100
  Discrete Derivative : simulink/Discrete/Discrete Derivative  gainval=1.0  ICPrevScaledInput=0.0  OutMin=[]  OutMax=[]  OutDataType=fixdt(1, 16)  OutScaling=2^-10  DoSatur=off
  Discrete-Time Integrator : DiscreteIntegrator  InitialConditionSetting=State (most efficient)  SampleTime=-1  LimitOutput=on  UpperSaturationLimit=Saturation_I_Y_Max  LowerSaturationLimit=Saturation_I_Y_Min  ICPrevOutput=DiscIntNeverNeededParam  ICPrevScaledInput=DiscIntNeverNeededParam
  Gain : Gain  Gain=Kp_YAW_AngleRate
  Integral Gain : Gain  DisableCoverage=on  Gain=Ki_YAW_AngleRate
  Sum : Sum  Inputs=+++
  y : Outport  InitialOutput=0
  wires:
  x/1 -> Gain/1, Integral Gain/1, Derivative Gain/1
  Integral Gain/1 -> Discrete-Time Integrator/1
  Derivative Gain/1 -> Discrete Derivative/1
  Gain/1 -> Sum/1
  Sum/1 -> y/1
  Discrete Derivative/1 -> Sum/3
  Discrete-Time Integrator/1 -> Sum/2

== system PosControl_Sim/Control System/Control System/AttitudeControl/P_pitch  ==
  x : Inport
  Gain : Gain  Gain=Kp_PITCH_ANGLE
  y : Outport  InitialOutput=0
  wires:
  x/1 -> Gain/1
  Gain/1 -> y/1

== system PosControl_Sim/Control System/Control System/AttitudeControl/P_roll  ==
  x : Inport
  Gain : Gain  Gain=Kp_ROLL_ANGLE
  y : Outport  InitialOutput=0
  wires:
  Gain/1 -> y/1
  x/1 -> Gain/1

== system PosControl_Sim/Control System/Control System/position_control/px ==
  ex : Inport
  Gain1 : Gain  Gain=Kpxp
  Saturation3 : Saturate  UpperLimit=MAX_CONTROL_VELOCITY_XY  LowerLimit=-MAX_CONTROL_VELOCITY_XY
  vxd : Outport
  wires:
  ex/1 -> Gain1/1
  Saturation3/1 -> vxd/1
  Gain1/1 -> Saturation3/1

== system PosControl_Sim/Control System/Control System/position_control/py ==
  ey : Inport
  Gain1 : Gain  Gain=Kpyp
  Saturation3 : Saturate  UpperLimit=MAX_CONTROL_VELOCITY_XY  LowerLimit=-MAX_CONTROL_VELOCITY_XY
  vyd : Outport
  wires:
  Gain1/1 -> Saturation3/1
  Saturation3/1 -> vyd/1
  ey/1 -> Gain1/1

== system PosControl_Sim/Control System/Control System/position_control/pz ==
  ez : Inport
  Gain1 : Gain  Gain=Kpzp
  Saturation3 : Saturate  UpperLimit=MAX_CONTROL_VELOCITY_Z  LowerLimit=-MAX_CONTROL_VELOCITY_Z
  vzd : Outport
  wires:
  ez/1 -> Gain1/1
  Saturation3/1 -> vzd/1
  Gain1/1 -> Saturation3/1

== system PosControl_Sim/Control System/Control System/position_control/vx  ==
  x : Inport
  Derivative Gain : Gain  DisableCoverage=on  Gain=Kvxd
  Discrete Derivative : simulink/Discrete/Discrete Derivative  gainval=1.0  ICPrevScaledInput=0.0  OutMin=[]  OutMax=[]  OutDataType=fixdt(1, 16)  OutScaling=2^-10  DoSatur=off
  Discrete-Time Integrator : DiscreteIntegrator  InitialConditionSetting=State (most efficient)  SampleTime=-1  LimitOutput=on  UpperSaturationLimit=Saturation_I_ah  LowerSaturationLimit=-Saturation_I_ah  ICPrevOutput=DiscIntNeverNeededParam  ICPrevScaledInput=DiscIntNeverNeededParam
  Gain : Gain  Gain=Kvxp
  Integral Gain : Gain  DisableCoverage=on  Gain=Kvxi
  Sum : Sum  Inputs=+++
  y : Outport  InitialOutput=0
  wires:
  x/1 -> Gain/1, Integral Gain/1, Derivative Gain/1
  Integral Gain/1 -> Discrete-Time Integrator/1
  Derivative Gain/1 -> Discrete Derivative/1
  Gain/1 -> Sum/1
  Sum/1 -> y/1
  Discrete Derivative/1 -> Sum/3
  Discrete-Time Integrator/1 -> Sum/2

== system PosControl_Sim/Control System/Control System/position_control/vy  ==
  x : Inport
  Derivative Gain : Gain  DisableCoverage=on  Gain=Kvyd
  Discrete Derivative : simulink/Discrete/Discrete Derivative  gainval=1.0  ICPrevScaledInput=0.0  OutMin=-5  OutMax=5  OutDataType=fixdt(1, 16)  OutScaling=2^-10  DoSatur=off
  Discrete-Time Integrator : DiscreteIntegrator  InitialConditionSetting=State (most efficient)  SampleTime=-1  LimitOutput=on  UpperSaturationLimit=Saturation_I_ah  LowerSaturationLimit=-Saturation_I_ah  ICPrevOutput=DiscIntNeverNeededParam  ICPrevScaledInput=DiscIntNeverNeededParam
  Gain : Gain  Gain=Kvyp
  Integral Gain : Gain  DisableCoverage=on  Gain=Kvyi
  Sum : Sum  Inputs=+++  OutMin=-5  OutMax=5
  y : Outport  InitialOutput=0
  wires:
  x/1 -> Gain/1, Integral Gain/1, Derivative Gain/1
  Integral Gain/1 -> Discrete-Time Integrator/1
  Derivative Gain/1 -> Discrete Derivative/1
  Gain/1 -> Sum/1
  Sum/1 -> y/1
  Discrete Derivative/1 -> Sum/3
  Discrete-Time Integrator/1 -> Sum/2

== system PosControl_Sim/Control System/Control System/position_control/vz  ==
  x : Inport
  Derivative Gain : Gain  DisableCoverage=on  Gain=Kvzd
  Discrete Derivative : simulink/Discrete/Discrete Derivative  gainval=1.0  ICPrevScaledInput=0.0  OutMin=[]  OutMax=[]  OutDataType=fixdt(1, 16)  OutScaling=2^-10  DoSatur=off
  Discrete-Time Integrator : DiscreteIntegrator  InitialConditionSetting=State (most efficient)  SampleTime=-1  LimitOutput=on  UpperSaturationLimit=Saturation_I_az  LowerSaturationLimit=-Saturation_I_az  ICPrevOutput=DiscIntNeverNeededParam  ICPrevScaledInput=DiscIntNeverNeededParam
  Gain : Gain  Gain=Kvzp
  Integral Gain : Gain  DisableCoverage=on  Gain=Kvzi
  Sum : Sum  Inputs=+++
  y : Outport  InitialOutput=0
  wires:
  Discrete-Time Integrator/1 -> Sum/2
  Discrete Derivative/1 -> Sum/3
  Sum/1 -> y/1
  Gain/1 -> Sum/1
  Derivative Gain/1 -> Discrete Derivative/1
  Integral Gain/1 -> Discrete-Time Integrator/1
  x/1 -> Derivative Gain/1, Integral Gain/1, Gain/1

== system PosControl_Sim/Quadcopter Dynamics simplified /刚体模型/刚体动力学模型/J*w ==
  p q r : Inport
  J : Inport  Port=2
  J*w : Product  Multiplication=Matrix(*)
  "J*w " : Outport
  wires:
  p q r/1 -> J*w/2
  J/1 -> J*w/1
  J*w/1 -> "J*w "/1

== matlab function PosControl_Sim/Control System/InputConditioning/deadzone ==
  data: u input; y output
function y = fcn(u)
%将遥控输入的范围控制在1100~1900，同时设置一个死区，死区大小为±deadZone
RCMin = 1100;
RCMax = 1900;
RCMid = (RCMin+RCMax)/2;
deadZoneRate = 0.02;
deadZone = deadZoneRate*(RCMax-RCMin);
k=1/(RCMax-RCMid-deadZone);
%限幅
if(u < RCMin)
    u = RCMin;
elseif(u > RCMax)
    u = RCMax;
end
%死区
 if(u > RCMid+deadZone)
    y = (u-RCMid-deadZone)*k;
 elseif(u < RCMid-deadZone)
     y = (u-RCMid+deadZone)*k;
 else
     y = 0;
 end

 end

== matlab function PosControl_Sim/Control System/InputConditioning/deadzone1 ==
  data: u input; y output
function y = fcn(u)
%将遥控输入的范围控制在1100~1900，同时设置一个死区，死区大小为±deadZone
RCMin = 1100;
RCMax = 1900;
RCMid = (RCMin+RCMax)/2;
deadZoneRate = 0.05;
deadZone = deadZoneRate*(RCMax-RCMin);
k=1/(RCMax-RCMid-deadZone);
%限幅
if(u < RCMin)
    u = RCMin;
elseif(u > RCMax)
    u = RCMax;
end
%死区
 if(u > RCMid+deadZone)
    y = (u-RCMid-deadZone)*k;
 elseif(u < RCMid-deadZone)
     y = (u-RCMid+deadZone)*k;
 else
     y = 0;
 end

 end

== matlab function PosControl_Sim/Control System/InputConditioning/deadzone2 ==
  data: u input; y output
function y = fcn(u)
%将遥控输入的范围控制在1100~1900，同时设置一个死区，死区大小为±deadZone
RCMin = 1100;
RCMax = 1900;
RCMid = (RCMin+RCMax)/2;
deadZoneRate = 0.05;
deadZone = deadZoneRate*(RCMax-RCMin);
k=1/(RCMax-RCMid-deadZone);
%限幅
if(u < RCMin)
    u = RCMin;
elseif(u > RCMax)
    u = RCMax;
end
%死区
 if(u > RCMid+deadZone)
    y = (u-RCMid-deadZone)*k;
 elseif(u < RCMid-deadZone)
     y = (u-RCMid+deadZone)*k;
 else
     y = 0;
 end

 end

== matlab function PosControl_Sim/Control System/InputConditioning/deadzone3 ==
  data: u input; y output
function y = fcn(u)
%将遥控输入的范围控制在1100~1900，同时设置一个死区，死区大小为±deadZone
RCMin = 1100;
RCMax = 1900;
RCMid = (RCMin+RCMax)/2;
deadZoneRate = 0.05;
deadZone = deadZoneRate*(RCMax-RCMin);
k=1/(RCMax-RCMid-deadZone);
%限幅
if(u < RCMin)
    u = RCMin;
elseif(u > RCMax)
    u = RCMax;
end
%死区
 if(u > RCMid+deadZone)
    y = (u-RCMid-deadZone)*k;
 elseif(u < RCMid-deadZone)
     y = (u-RCMid+deadZone)*k;
 else
     y = 0;
 end

 end

== matlab function PosControl_Sim/Control System/Control System/position_control/MATLAB Function ==
  data: eax input; eay input; psi input; phi output; theta output
function [phi,theta] = fcn(eax,eay,psi)
g=9.8;
phi = (-sin(psi)*eax + cos(psi)*eay)/g;
theta = (-cos(psi)*eax-sin(psi)*eay)/g;

== matlab function PosControl_Sim/Control System/Control System/pwm_out2 ==
  data: Roll input; M1 output; Pitch input; Yaw input; Thrust input; M2 output; M3 output; M4 output
function [M1, M2, M3, M4] = motor_mixer(Roll, Pitch, Yaw, Thrust)
%quadrotorX
%3     1
%  \ /
%  / \
%2     4

idle_PWM = 1000;
scale = 1000;

M1 = (Thrust - Roll + Pitch + Yaw) * scale + idle_PWM;
M2 = (Thrust + Roll - Pitch + Yaw) * scale + idle_PWM;
M3 = (Thrust + Roll + Pitch - Yaw) * scale + idle_PWM;
M4 = (Thrust - Roll - Pitch - Yaw) * scale + idle_PWM;

== matlab function PosControl_Sim/Quadcopter Dynamics simplified /刚体模型/刚体动力学模型/陀螺力矩 ==
  data: Jrp input; MotorRads input; pqr input; Ga output
function Ga = fcn(Jrp,MotorRads,pqr)
Ga=zeros(3,1);
Ga(1)=Jrp*pqr(2)*(-MotorRads(1)-MotorRads(2)+MotorRads(3)+MotorRads(4));
Ga(2)=Jrp*pqr(1)*( MotorRads(1)+MotorRads(2)-MotorRads(3)-MotorRads(4));

== matlab function PosControl_Sim/Quadcopter Dynamics simplified /刚体模型/计算旋转矩阵和欧拉角/四元数转欧拉角 ==
  data: q input; y output
function y = fcn(q)
Rbe = [q(1)*q(1) + q(2)*q(2) - q(3)*q(3) - q(4)*q(4), 2*(q(2)*q(3) - q(1)*q(4)), 2*(q(2)*q(4) + q(1)*q(3))
       2*(q(2)*q(3) + q(1)*q(4)), q(1)*q(1) - q(2)*q(2) + q(3)*q(3) - q(4)*q(4), 2*(q(3)*q(4) - q(1)*q(2))
       2*(q(2)*q(4) - q(1)*q(3)), 2*(q(3)*q(4) + q(1)*q(2)), q(1)*q(1) - q(2)*q(2) - q(3)*q(3) + q(4)*q(4)];
   
phi = atan2(Rbe(3,2),Rbe(3,3));
theta = asin(-Rbe(3,1));
psi = atan2(Rbe(2,1),Rbe(1,1));  
% phi = atan2(2*(q(1)*q(2)+q(3)*q(4)),(1-2*(q(2)*q(2)+q(3)*q(3))));
% theta = asin(2*(q(1)*q(3)-q(2)*q(4)));
% psi = atan2(2*(q(1)*q(4)+q(2)*q(3)),(1-2*(q(3)*q(3))+q(4)*q(4)));
y = [phi theta psi];

== matlab function PosControl_Sim/Quadcopter Dynamics simplified /刚体模型/计算旋转矩阵和欧拉角/基于四元数模型 ==
  data: pqr input; qdot output; q input
function qdot = fcn(pqr,q)

qdot=0.5*[0,-pqr(1),-pqr(2),-pqr(3);pqr(1),0,pqr(3),-pqr(2);pqr(2),-pqr(3),0,pqr(1);pqr(3),pqr(2),-pqr(1),0]*q;

== matlab function PosControl_Sim/Quadcopter Dynamics simplified /控制效率模型/Propeller Model ==
  data: w input; R input; Fb output; Fd output; Mb output; Cm input; Ct input; Vb input; Cd input
function [Fb,Fd,Mb] = fcn(w,R,Cm,Ct,Vb,Cd)
 %%叉字型
 %3  1
 %2  4
 M_rctcm = [-sin(pi/4)*R*Ct,sin(pi/4)*R*Ct,sin(pi/4)*R*Ct,-sin(pi/4)*R*Ct;
            sin(pi/4)*R*Ct,-sin(pi/4)*R*Ct,sin(pi/4)*R*Ct,-sin(pi/4)*R*Ct;
            Cm,Cm,-Cm,-Cm];
 Mb = M_rctcm*(w.^2);%式(6.24),力矩
 
 Fb = [0; 0; -sum(Ct*(w.^2))]; %(6.23),螺旋桨拉力
 Fd = -Cd*Vb.*abs(Vb)*0.5;%空气阻力
end

== matlab function PosControl_Sim/Control System/MATLAB Function ==
  data: vx_d output; vy_d output; vz_d output; vxd input; vyd input; vzd input; x input; y input; x_d output; y_d output; z input; z_d output
function [vx_d,vy_d,vz_d,x_d,y_d,z_d]  = fcn(vxd,vyd,vzd,x,y,z)

persistent x1;
if isempty(x1)
    x1=0;
end
persistent y1;
if isempty(y1)
    y1=0;
end
persistent z1;
if isempty(z1)
    z1=z;
end
persistent hold_x_flag;
if isempty(hold_x_flag)
    hold_x_flag=0;
end
persistent hold_y_flag;
if isempty(hold_y_flag)
    hold_y_flag=0;
end
persistent hold_z_flag;
if isempty(hold_z_flag)
    hold_z_flag=0;
end
if abs(vxd)<0.001
    hold_x=1;
else
    hold_x=0;
end
if abs(vyd)<0.001
    hold_y=1;
else
    hold_y=0;
end
if abs(vzd)<0.001
    hold_z=1;
else
    hold_z=0;
end

%摇杆在中间，保持位置
if (hold_x>0.5)&&(hold_x_flag<0.5)
    x1=x;
    hold_x_flag=1;
end
if (hold_y>0.5)&&(hold_y_flag<0.5)
    y1=y;
    hold_y_flag=1;
end
%油门在中间位置，保持高度
if (hold_z>0.5)&&(hold_z_flag<0.5)
    z1=z;
    hold_z_flag=1;
end

if hold_x<0.5
    x1=x;
    hold_x_flag = 0;
end
if hold_y<0.5
    y1=y;
    hold_y_flag = 0;
end
%油门不在中间位置，期望高度即为当前高度。高度控制器只有速度环起作用
if hold_z<0.5
    z1=z;
    hold_z_flag = 0;
end

vx_d=vxd;vy_d=vyd;vz_d=vzd;
x_d=x1;
y_d=y1;
z_d=z1;
